simulink model "step10_observer"  (R2025a)
settings: Solver=ode45  StartTime=0.0  StopTime=20  MaxStep=0.01  RelTol=1e-3
undefined symbols (not defined in the file or in its folder): A, B, F, K, L
libraries: SignalEditorBlockLib x1
settings Model: Creator=O M E N  LastModifiedBy=O M E N

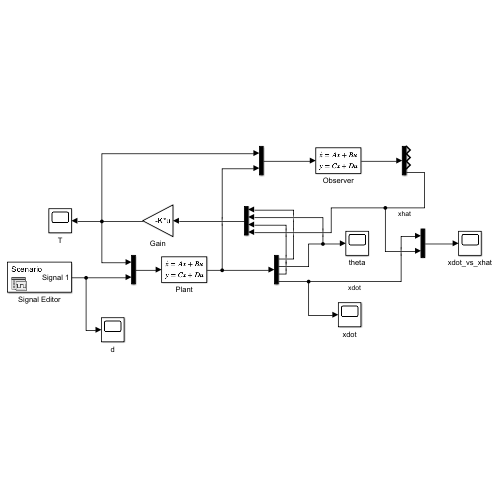
[thumbnail: Simulink's stored preview of the top-level diagram]
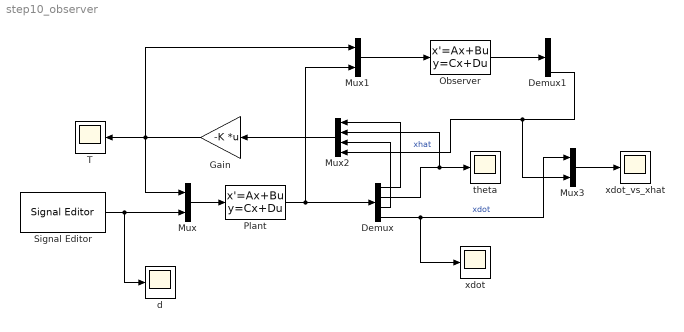
== system step10_observer ==
  Demux : Demux
  Demux1 : Demux
  Gain : Gain  Gain=-K  Multiplication=Matrix(K*u)
  Mux : Mux  Inputs=2
  Mux1 : Mux  Inputs=2
  Mux2 : Mux
  Mux3 : Mux  Inputs=2
  Observer : StateSpace  A=A - L  B=[B L]  C=eye(4)  D=zeros(4,5)  InitialCondition=[0; 0; 0; 0.05]
  Plant : StateSpace  A=A  B=[B F]  C=eye(4)  D=zeros(4,2)  InitialCondition=[0; 0; 0; 0]
  Signal Editor : SignalEditorBlockLib/Signal Editor  FileName=d_trapezoid.mat  ActiveScenario=Scenario  ActiveSignal=Signal 1  IsBus=off  OutputBusObjectStr=Bus: BusObject  SampleTime=0  ZeroCross=off  OutputAfterFinalValue=Setting to zero  Unit=inherit  PreserveSignalName=on  ApplySigPropsToAllScenarios=on  ApplySigPropsToAllSignals=off  SignalPropertySource=Dialog parameters
  T : Scope
      settings: Title=Control torque T(t)  ActiveDisplayYMinimum=-1  ActiveDisplayYMaximum=1  YLabel="T  (N·m)"  DataLoggingVariableName=ScopeData2
  d : Scope
      settings: Title=Disturbance d(t)  ActiveDisplayYMinimum=-0.0012499999999999998  ActiveDisplayYMaximum=0.01125  YLabel="d  (m)"  DataLoggingVariableName=ScopeData3
  theta : Scope
      settings: Title=Tilt angle θ(t)  ActiveDisplayYMinimum=-1  ActiveDisplayYMaximum=1  YLabel="θ  (rad)"
  xdot : Scope
      settings: Title=Vehicle speed ẋ(t)  ActiveDisplayYMinimum=-1  ActiveDisplayYMaximum=1  YLabel="ẋ  (m/s)"
  xdot_vs_xhat : Scope
      settings: Title=True vs. estimated speed  ActiveDisplayYMinimum=-1.0012810447181375  ActiveDisplayYMaximum=3.1244086781731943  YLabel="ẋ, ẋ̂  (m/s)"  DataLoggingVariableName=ScopeData4
  wires:
  Mux/1 -> Plant/1
  Plant/1 -> Demux/1, Mux1/2
  Demux/2 -> Mux2/2, theta/1
  Demux/4 -> Mux3/1, xdot/1  "xdot"
  Gain/1 -> Mux1/1, T/1, Mux/1
  Signal Editor/1 -> d/1, Mux/2
  Mux1/1 -> Observer/1
  Observer/1 -> Demux1/1
  Demux/1 -> Mux2/1
  Demux/3 -> Mux2/3
  Demux1/4 -> Mux2/4, Mux3/2  "xhat"
  Mux2/1 -> Gain/1
  Mux3/1 -> xdot_vs_xhat/1
